simulink model "kr2_sim"  (Simulink 7.5)
settings: Solver=ode45  StartTime=0.0  StopTime=6.3  RelTol=1e-3
settings Model: Creator=Dranik_win  LastModifiedBy=Dranik_win

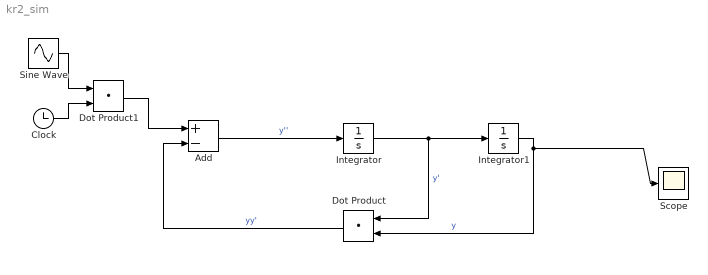
== system kr2_sim ==
  Add : Sum  Inputs=+-  OutDataType=fixdt(1, 16)  OutScaling=2^-10
  Clock : Clock
      settings: Decimation=10
  Dot Product : DotProduct  OutDataType=fixdt(1, 16)  OutScaling=2^-10  InputSameDT=on  OutDataTypeStr=Inherit: Inherit via internal rule
  Dot Product1 : DotProduct  OutDataType=fixdt(1, 16)  OutScaling=2^-10  InputSameDT=on  OutDataTypeStr=Inherit: Inherit via internal rule
  Integrator : Integrator
  Integrator1 : Integrator  InitialCondition=1
  Scope : Scope
  Sine Wave : Sin  Amplitude=1  Bias=0  Frequency=1  Phase=0  Samples=10  SampleTime=0  Offset=0
  wires:
  Integrator/1 -> Integrator1/1, Dot Product/1  "y'"
  Integrator1/1 -> Dot Product/2, Scope/1  "y"
  Dot Product/1 -> Add/2  "yy'"
  Add/1 -> Integrator/1  "y''"
  Sine Wave/1 -> Dot Product1/1
  Clock/1 -> Dot Product1/2
  Dot Product1/1 -> Add/1
